simulink model "es1_2"  (R2014a)
settings: Solver=ode45  StartTime=0.0  StopTime=20  RelTol=1e-3
values from neighbouring files (symbols this model uses):
  Kc = 800    [es1.m]
  Kr = 2    [es1.m]
libraries: cstblocks x1, simulink x1
settings Model: Creator=HP  LastModifiedBy=HP

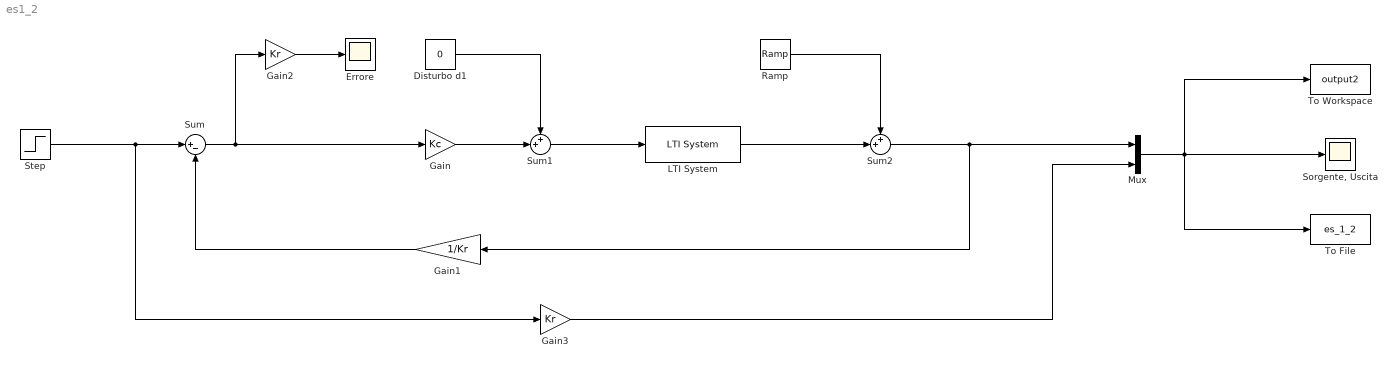
== system es1_2 ==
  Disturbo d1 : Constant  Value=0
  Errore : Scope
      settings: MaxDataPoints=50000
  Gain : Gain  Gain=Kc
  Gain1 : Gain  Gain=1/Kr
  Gain2 : Gain  Gain=Kr
  Gain3 : Gain  Gain=Kr
  LTI System : cstblocks/LTI System  sys=F  IC=[]
  Mux : Mux  Inputs=2
  Ramp : simulink/Sources/Ramp  slope=0.01  start=0  X0=0
  "Sorgente, Uscita" : Scope
      settings: MaxDataPoints=50000
  Step : Step  Time=0  After=2  SampleTime=0
  Sum : Sum  Inputs=|+-
  Sum1 : Sum  Inputs=++|
  Sum2 : Sum  Inputs=++|
  To File : ToFile  Filename=es_1_2  SaveFormat=Timeseries
  To Workspace : ToWorkspace  VariableName=output2  SaveFormat=Timeseries  SampleTime=-1
  wires:
  Step/1 -> Gain3/1, Sum/1
  Gain1/1 -> Sum/2
  Sum/1 -> Gain2/1, Gain/1
  Gain2/1 -> Errore/1
  Disturbo d1/1 -> Sum1/1
  Gain/1 -> Sum1/2
  Sum1/1 -> LTI System/1
  Ramp/1 -> Sum2/1
  LTI System/1 -> Sum2/2
  Mux/1 -> To Workspace/1, To File/1, "Sorgente, Uscita"/1
  Sum2/1 -> Gain1/1, Mux/1
  Gain3/1 -> Mux/2
